simulink model "state_space"  (R2021b)
settings: Solver=VariableStepAuto  StartTime=0.0  StopTime=20.0  RelTol=1e-3
values from neighbouring files (symbols this model uses):
  A = [0      1              0           0 ... (first row only)    [system_modelling.m]
  B = [     0 ... (first row only)    [system_modelling.m]
  C = [1 0 0 0 ... (first row only)    [system_modelling.m]
  k_matrix = Klqr    [system_modelling.m]
  x_ref = [0.3 ... (first row only)    [system_modelling.m]
settings Model: Creator=91725  LastModifiedBy=91725

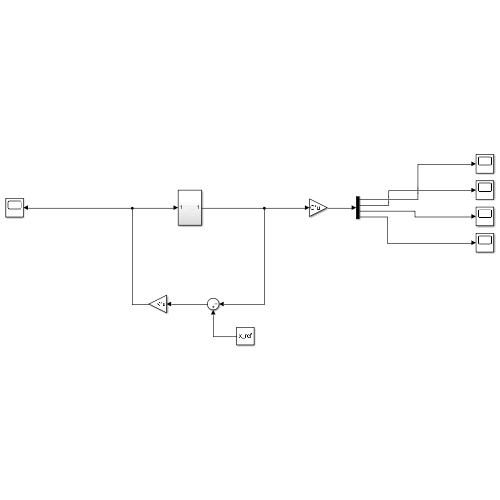
[thumbnail: Simulink's stored preview of the top-level diagram]
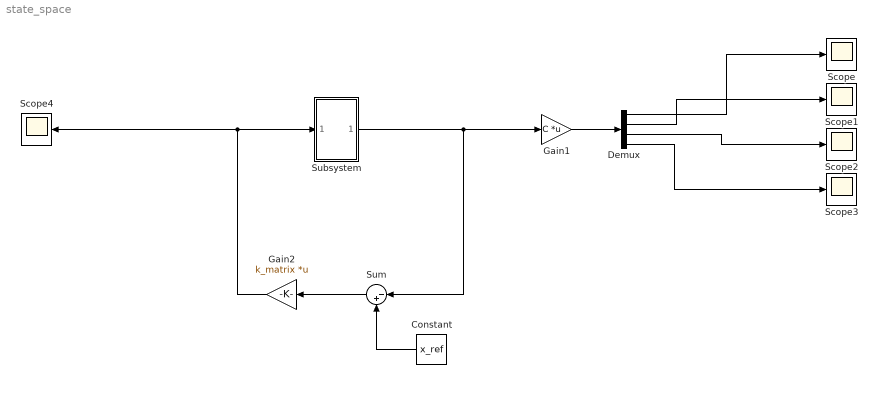
== system state_space ==
  Constant : Constant  Value=x_ref
  Demux : Demux
  Gain1 : Gain  Gain=C  Multiplication=Matrix(K*u)
  Gain2 : Gain  Gain=k_matrix  Multiplication=Matrix(K*u)
  Scope{,1..4} (5 alike) : Scope
  Subsystem : Subsystem
  Sum : Sum  Inputs=|-+
  wires:
  Subsystem/1(Out1) -> Sum/1, Gain1/1
  Constant/1 -> Sum/2
  Sum/1 -> Gain2/1
  Gain1/1 -> Demux/1
  Demux/1 -> Scope/1
  Demux/2 -> Scope1/1
  Demux/3 -> Scope2/1
  Demux/4 -> Scope3/1
  Gain2/1 -> Subsystem/1(In1), Scope4/1

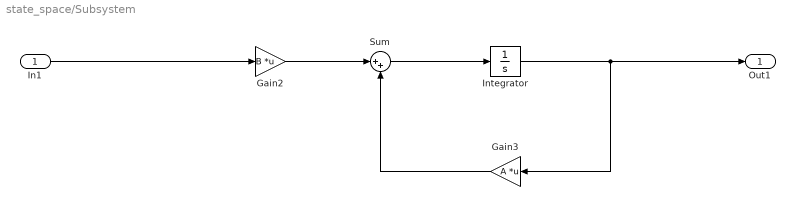
== system state_space/Subsystem ==
  In1 : Inport
  Gain2 : Gain  Gain=B  Multiplication=Matrix(K*u)
  Gain3 : Gain  Gain=A  Multiplication=Matrix(K*u)
  Integrator : Integrator
  Sum : Sum  Inputs=|++
  Out1 : Outport
  wires:
  Integrator/1 -> Out1/1, Gain3/1
  Gain3/1 -> Sum/2
  Sum/1 -> Integrator/1
  Gain2/1 -> Sum/1
  In1/1 -> Gain2/1
